simulink model "propeller"  (R2019b)
settings: Solver=VariableStepAuto  StartTime=0.0  StopTime=180  MaxStep=1e-2  RelTol=1e-3
undefined symbols (not defined in the file or in its folder): X, Y, Z
libraries: sm_lib x26, cstblocks x23, nesl_utility x20, simulink x2
(part 3 of 3)

== system propeller/直接转矩控制/船速、朝向控制器/推力解算/扭矩有解 ==
  状态输入 : Inport
  Action Port : ActionPort  ActionPortLabel=else
  If : If
  If Action Subsystem : Subsystem  TreatAsAtomicUnit=on
  If Action Subsystem1 : Subsystem  TreatAsAtomicUnit=on
  Merge : Merge
  通解选择 : Fcn  Expr=abs(u(5)+u(3)) - abs(u(5)-u(4))
  推力输出 : Outport
  wires:
  If Action Subsystem/1(推力) -> Merge/1
  If/1 -> If Action Subsystem/Action
  状态输入/1 -> If Action Subsystem1/1(In1), 通解选择/1, If Action Subsystem/1(In1)
  通解选择/1 -> If/1
  If Action Subsystem1/1(推力) -> Merge/2
  If/2 -> If Action Subsystem1/Action
  Merge/1 -> 推力输出/1  "推力输出"

== system propeller/直接转矩控制/船速、朝向控制器/舵内缩指令/If Action Subsystem ==
  Action Port : ActionPort  ActionPortLabel=else
  Constant : Constant  Value=0
  Out1 : Outport
  wires:
  Constant/1 -> Out1/1

== system propeller/直接转矩控制/船速、朝向控制器/舵内缩指令/Subsystem ==
  前进力 : Inport
  转向扭矩 : Inport  Port=2
  Action Port : ActionPort  ActionPortLabel=if(u1 < 0)
  Constant : Constant  Value=Trq_Start
  Gain : Gain  Gain=0.5
  Gain1 : Gain  Gain=0.1
  Gain2 : Gain  Gain=-1
  Integrator : Integrator  LimitOutput=on  UpperSaturationLimit=Th_Max*2  LowerSaturationLimit=0
  Mux : Mux  Inputs=2
  Sum : Sum  Inputs=|+-
  Sum3 : Sum  Inputs=|+-
  收敛用推力解算 : Subsystem  mask{a=1, b=3}
      mask prompts: a "推进器安装横向距离 a"; b "推进器安装纵向距离 b"
  左右差 : Outport
  wires:
  转向扭矩/1 -> 收敛用推力解算/2(转向扭矩)
  收敛用推力解算/1(左推力) -> Sum3/1
  Mux/1 -> 收敛用推力解算/3(左右推进偏角)
  Sum3/1 -> Sum/1
  前进力/1 -> 收敛用推力解算/1(前进力)
  Integrator/1 -> Gain/1, 左右差/1
  Gain/1 -> Gain2/1, Mux/1
  收敛用推力解算/2(右推力) -> Sum3/2
  Gain2/1 -> Mux/2
  Constant/1 -> Sum/2
  Sum/1 -> Gain1/1
  Gain1/1 -> Integrator/1

== system propeller/直接转矩控制/船速、朝向控制器/舵朝向指令/If Action Subsystem ==
  Action Port : ActionPort  ActionPortLabel=else
  Constant : Constant  Value=0
  Out1 : Outport
  wires:
  Constant/1 -> Out1/1

== system propeller/直接转矩控制/船速、朝向控制器/舵朝向指令/Subsystem ==
  前进力 : Inport
  转向扭矩 : Inport  Port=2
  Action Port : ActionPort  ActionPortLabel=if(u1 > 0)
  Gain : Gain  Gain=0.5
  Gain1 : Gain  Gain=0.1
  Integrator : Integrator  LimitOutput=on  UpperSaturationLimit=Th_Max*2  LowerSaturationLimit=-Th_Max*2
  Mux : Mux  Inputs=2
  Sum3 : Sum  Inputs=|+-
  收敛用推力解算 : Subsystem  mask{a=1, b=3}
      mask prompts: a "推进器安装横向距离 a"; b "推进器安装纵向距离 b"
  左右和 : Outport
  wires:
  收敛用推力解算/2(右推力) -> Sum3/2
  Gain/1 -> Mux/1, Mux/2
  Integrator/1 -> 左右和/1, Gain/1
  前进力/1 -> 收敛用推力解算/1(前进力)
  Sum3/1 -> Gain1/1
  Gain1/1 -> Integrator/1
  Mux/1 -> 收敛用推力解算/3(左右推进偏角)
  收敛用推力解算/1(左推力) -> Sum3/1
  转向扭矩/1 -> 收敛用推力解算/2(转向扭矩)

== system propeller/直接转矩控制/船速、朝向控制器/船头方向PID/反馈量滤波 ==
  Signal : Inport
  Constant2 : Constant  Value=Frq
  Gain : Gain  Gain=2*pi
  d_Smp_LPF6 : cstblocks/Linear Parameter Varying/Varying Lowpass Filter  N=Order
      settings: SourceProductName=Control System Toolbox
  Output : Outport
  wires:
  Gain/1 -> d_Smp_LPF6/2
  Signal/1 -> d_Smp_LPF6/1
  Constant2/1 -> Gain/1
  d_Smp_LPF6/1 -> Output/1  "Is"

== system propeller/直接转矩控制/船速、朝向控制器/船头方向PID/微分 ==
  Err : Inport
  Derivative : Derivative  CoefficientInTFapproximation=0.1
  微分滤波1 : Subsystem  mask{Frq=fc_Set, Order=3}
      mask prompts: Frq "Frq_Set"; Order "Order_Set"
  dErr : Outport
  wires:
  Err/1 -> 微分滤波1/1(Signal)
  微分滤波1/1(Output) -> Derivative/1
  Derivative/1 -> dErr/1

== system propeller/直接转矩控制/船速、朝向控制器/船头方向PID/积分控制 ==
  note: 角度快速增大时积分不增大
      | 角度快速减小时积分不减小
  Error : Inport
  Output : Inport  Port=2
  Derivative : Derivative  CoefficientInTFapproximation=0.1
  Memory : Memory
  Memory1 : Memory
  Product1 : Product  Inputs=3
  Scope : Scope  NumInputPorts=3
  Subsystem : Subsystem
  Zero-Order Hold : ZeroOrderHold  SampleTime=0.01
  Zero-Order Hold1 : ZeroOrderHold  SampleTime=0.01
  Zero-Order Hold2 : ZeroOrderHold  SampleTime=0.01
  输出达到正限幅时积分不再增大 : Subsystem
  输出达到负限幅时积分不再减小 : Subsystem
  开启积分 : Outport
  wires:
  Memory1/1 -> 输出达到正限幅时积分不再增大/2(Out), 输出达到负限幅时积分不再减小/2(Out)
  Memory/1 -> Subsystem/2(Err), 输出达到负限幅时积分不再减小/1(Err), 输出达到正限幅时积分不再增大/1(Err)
  Error/1 -> Derivative/1, Zero-Order Hold/1
  Product1/1 -> 开启积分/1
  Output/1 -> Zero-Order Hold2/1
  输出达到负限幅时积分不再减小/1(启动积分) -> Scope/3, Product1/3  "负限幅限制"
  输出达到正限幅时积分不再增大/1(启动积分) -> Scope/2, Product1/2  "正限幅限制"
  Zero-Order Hold/1 -> Memory/1
  Derivative/1 -> Zero-Order Hold1/1
  Zero-Order Hold2/1 -> Memory1/1
  Zero-Order Hold1/1 -> Subsystem/1(dErr)
  Subsystem/1(启动积分) -> Scope/1, Product1/1  "斜率限制"

== system propeller/失败的水流估计模型/水流状态估计/螺旋桨状态模拟/螺旋桨工作特性表/If Action Subsystem2 ==
  J' : Inport
  Action Port : ActionPort  ActionPortLabel=if(u1 > 0)
  n+::Kq-扭矩系数 : Lookup_n-D  NumberOfTableDimensions=1  BreakpointsForDimension1=[-1,-0.9,-0.8,-0.7,-0.6,-0.5,-0.4,-0.3,-0.2,-0.1,0,0.1,0.2,0.3,0.4,0.5,0.6,0.7,0.8,0.9,1]  BreakpointsForDimension2=[1:3]  Table=[0.019242,0.038636,0.046717,0.049444,0.050032,0.050032,0.050291,0.05055,0.051327,0.051845,0.05197,0.050556,0.046111,0.040556,0.033081,0.024596,0.015543,0.0059848,-0.0059091,-0.013687,-0.016818]  InternalRulePriority=Speed  RndMeth=Simplest  InputSameDT=on
  n+::Kt-推力系数 : Lookup_n-D  NumberOfTableDimensions=1  BreakpointsForDimension1=[-1,-0.9,-0.8,-0.7,-0.6,-0.5,-0.4,-0.3,-0.2,-0.1,0,0.1,0.2,0.3,0.4,0.5,0.6,0.7,0.8,0.9,1]  BreakpointsForDimension2=[1:3]  Table=[0.082134,0.19766,0.30499,0.32898,0.33608,0.33932,0.34256,0.34741,0.36197,0.3738,0.38,0.36686,0.32645,0.26016,0.18188,0.10423,0.04173,-0.018245,-0.05423,-0.065593,-0.06]  InternalRulePriority=Speed  RndMeth=Simplest  InputSameDT=on
  Kt : Outport
  Kq : Outport  Port=2
  wires:
  J'/1 -> n+::Kt-推力系数/1, n+::Kq-扭矩系数/1
  n+::Kt-推力系数/1 -> Kt/1
  n+::Kq-扭矩系数/1 -> Kq/1

== system propeller/失败的水流估计模型/水流状态估计/螺旋桨状态模拟/螺旋桨工作特性表/If Action Subsystem3 ==
  J' : Inport
  Action Port : ActionPort  ActionPortLabel=else
  n-::Kq-扭矩系数 : Lookup_n-D  NumberOfTableDimensions=1  BreakpointsForDimension1=[-1,-0.9,-0.8,-0.7,-0.6,-0.5,-0.4,-0.3,-0.2,-0.1,0,0.1,0.2,0.3,0.4,0.5,0.6,0.7,0.8,0.9,1]  BreakpointsForDimension2=[1:3]  Table=[0.019242,0.016111,0.010354,-0.00035354,-0.014293,-0.025707,-0.034495,-0.041263,-0.046515,-0.051162,-0.05197,-0.051845,-0.051586,-0.051068,-0.051068,-0.050809,-0.050291,-0.048997,-0.045631,-0.038434,-0.016818]  InternalRulePriority=Speed  RndMeth=Simplest  InputSameDT=on
  n-::Kt-推力系数 : Lookup_n-D  NumberOfTableDimensions=1  BreakpointsForDimension1=[-1,-0.9,-0.8,-0.7,-0.6,-0.5,-0.4,-0.3,-0.2,-0.1,0,0.1,0.2,0.3,0.4,0.5,0.6,0.7,0.8,0.9,1]  BreakpointsForDimension2=[1:3]  Table=[0.082134,0.088952,0.080745,0.052336,-0.020896,-0.090341,-0.16989,-0.25764,-0.32014,-0.34981,-0.35874,-0.36197,-0.36036,-0.35874,-0.35388,-0.34741,-0.3377,-0.32197,-0.2947,-0.21894,-0.06]  InternalRulePriority=Speed  RndMeth=Simplest  InputSameDT=on
  Kt : Outport
  Kq : Outport  Port=2
  wires:
  n-::Kq-扭矩系数/1 -> Kq/1
  n-::Kt-推力系数/1 -> Kt/1
  J'/1 -> n-::Kt-推力系数/1, n-::Kq-扭矩系数/1

== system propeller/失败的水流估计模型/水流状态估计/螺旋桨状态模拟/螺旋桨工作特性表Backup/If Action Subsystem2 ==
  J' : Inport
  Action Port : ActionPort
  n+::Kq-扭矩系数 : Lookup_n-D  NumberOfTableDimensions=1  BreakpointsForDimension1=[-1,-0.9,-0.8,-0.7,-0.6,-0.5,-0.4,-0.3,-0.2,-0.1,0,0.1,0.2,0.3,0.4,0.5,0.6,0.7,0.8,0.9,1]  BreakpointsForDimension2=[1:3]  Table=[0.019242,0.038636,0.046717,0.049444,0.048333,0.043384,0.043081,0.045202,0.049242,0.051465,0.05197,0.050556,0.046111,0.040556,0.033081,0.024596,0.015543,0.0059848,-0.0059091,-0.013687,-0.016818]  InternalRulePriority=Speed  RndMeth=Simplest  InputSameDT=on
  n+::Kt-推力系数 : Lookup_n-D  NumberOfTableDimensions=1  BreakpointsForDimension1=[-1,-0.9,-0.8,-0.7,-0.6,-0.5,-0.4,-0.3,-0.2,-0.1,0,0.1,0.2,0.3,0.4,0.5,0.6,0.7,0.8,0.9,1]  BreakpointsForDimension2=[1:3]  Table=[0.082134,0.19766,0.30499,0.32898,0.31256,0.2589,0.25511,0.28226,0.35107,0.3738,0.38,0.36686,0.32645,0.26016,0.18188,0.10423,0.04173,-0.018245,-0.05423,-0.065593,-0.06]  InternalRulePriority=Speed  RndMeth=Simplest  InputSameDT=on
  Kt : Outport
  Kq : Outport  Port=2
  wires:
  n+::Kq-扭矩系数/1 -> Kq/1
  n+::Kt-推力系数/1 -> Kt/1
  J'/1 -> n+::Kq-扭矩系数/1, n+::Kt-推力系数/1

== system propeller/失败的水流估计模型/水流状态估计/螺旋桨状态模拟/螺旋桨工作特性表Backup/If Action Subsystem3 ==
  J' : Inport
  Action Port : ActionPort
  n-::Kq-扭矩系数 : Lookup_n-D  NumberOfTableDimensions=1  BreakpointsForDimension1=[-1,-0.9,-0.8,-0.7,-0.6,-0.5,-0.4,-0.3,-0.2,-0.1,0,0.1,0.2,0.3,0.4,0.5,0.6,0.7,0.8,0.9,1]  BreakpointsForDimension2=[1:3]  Table=[0.019242,0.016111,0.010354,-0.00035354,-0.014293,-0.025707,-0.034495,-0.041263,-0.046515,-0.051162,-0.05197,-0.051465,-0.049242,-0.045202,-0.043081,-0.043384,-0.04702,-0.049343,-0.045909,-0.038434,-0.016818]  InternalRulePriority=Speed  RndMeth=Simplest  InputSameDT=on
  n-::Kt-推力系数 : Lookup_n-D  NumberOfTableDimensions=1  BreakpointsForDimension1=[-1,-0.9,-0.8,-0.7,-0.6,-0.5,-0.4,-0.3,-0.2,-0.1,0,0.1,0.2,0.3,0.4,0.5,0.6,0.7,0.8,0.9,1]  BreakpointsForDimension2=[1:3]  Table=[0.082134,0.088952,0.080745,0.052336,-0.020896,-0.090341,-0.16989,-0.25764,-0.32014,-0.34981,-0.35676,-0.35549,-0.33409,-0.29015,-0.25379,-0.24924,-0.30379,-0.32197,-0.2947,-0.21894,-0.06]  InternalRulePriority=Speed  RndMeth=Simplest  InputSameDT=on
  Kt : Outport
  Kq : Outport  Port=2
  wires:
  J'/1 -> n-::Kq-扭矩系数/1, n-::Kt-推力系数/1
  n-::Kt-推力系数/1 -> Kt/1
  n-::Kq-扭矩系数/1 -> Kq/1

== system propeller/失败的水流估计模型/预期转速计算/螺旋桨状态模拟/螺旋桨工作特性表/If Action Subsystem2 ==
  J' : Inport
  Action Port : ActionPort  ActionPortLabel=if(u1 > 0)
  n+::Kq-扭矩系数 : Lookup_n-D  NumberOfTableDimensions=1  BreakpointsForDimension1=[-1,-0.9,-0.8,-0.7,-0.6,-0.5,-0.4,-0.3,-0.2,-0.1,0,0.1,0.2,0.3,0.4,0.5,0.6,0.7,0.8,0.9,1]  BreakpointsForDimension2=[1:3]  Table=[0.019242,0.038636,0.046717,0.049444,0.050032,0.050032,0.050291,0.05055,0.051327,0.051845,0.05197,0.050556,0.046111,0.040556,0.033081,0.024596,0.015543,0.0059848,-0.0059091,-0.013687,-0.016818]  InternalRulePriority=Speed  RndMeth=Simplest  InputSameDT=on
  n+::Kt-推力系数 : Lookup_n-D  NumberOfTableDimensions=1  BreakpointsForDimension1=[-1,-0.9,-0.8,-0.7,-0.6,-0.5,-0.4,-0.3,-0.2,-0.1,0,0.1,0.2,0.3,0.4,0.5,0.6,0.7,0.8,0.9,1]  BreakpointsForDimension2=[1:3]  Table=[0.082134,0.19766,0.30499,0.32898,0.33608,0.33932,0.34256,0.34741,0.36197,0.3738,0.38,0.36686,0.32645,0.26016,0.18188,0.10423,0.04173,-0.018245,-0.05423,-0.065593,-0.06]  InternalRulePriority=Speed  RndMeth=Simplest  InputSameDT=on
  Kt : Outport
  Kq : Outport  Port=2
  wires:
  J'/1 -> n+::Kt-推力系数/1, n+::Kq-扭矩系数/1
  n+::Kt-推力系数/1 -> Kt/1
  n+::Kq-扭矩系数/1 -> Kq/1

== system propeller/失败的水流估计模型/预期转速计算/螺旋桨状态模拟/螺旋桨工作特性表/If Action Subsystem3 ==
  J' : Inport
  Action Port : ActionPort  ActionPortLabel=else
  n-::Kq-扭矩系数 : Lookup_n-D  NumberOfTableDimensions=1  BreakpointsForDimension1=[-1,-0.9,-0.8,-0.7,-0.6,-0.5,-0.4,-0.3,-0.2,-0.1,0,0.1,0.2,0.3,0.4,0.5,0.6,0.7,0.8,0.9,1]  BreakpointsForDimension2=[1:3]  Table=[0.019242,0.016111,0.010354,-0.00035354,-0.014293,-0.025707,-0.034495,-0.041263,-0.046515,-0.051162,-0.05197,-0.051845,-0.051586,-0.051068,-0.051068,-0.050809,-0.050291,-0.048997,-0.045631,-0.038434,-0.016818]  InternalRulePriority=Speed  RndMeth=Simplest  InputSameDT=on
  n-::Kt-推力系数 : Lookup_n-D  NumberOfTableDimensions=1  BreakpointsForDimension1=[-1,-0.9,-0.8,-0.7,-0.6,-0.5,-0.4,-0.3,-0.2,-0.1,0,0.1,0.2,0.3,0.4,0.5,0.6,0.7,0.8,0.9,1]  BreakpointsForDimension2=[1:3]  Table=[0.082134,0.088952,0.080745,0.052336,-0.020896,-0.090341,-0.16989,-0.25764,-0.32014,-0.34981,-0.35874,-0.36197,-0.36036,-0.35874,-0.35388,-0.34741,-0.3377,-0.32197,-0.2947,-0.21894,-0.06]  InternalRulePriority=Speed  RndMeth=Simplest  InputSameDT=on
  Kt : Outport
  Kq : Outport  Port=2
  wires:
  n-::Kq-扭矩系数/1 -> Kq/1
  n-::Kt-推力系数/1 -> Kt/1
  J'/1 -> n-::Kt-推力系数/1, n-::Kq-扭矩系数/1

== system propeller/失败的水流估计模型/预期转速计算/螺旋桨状态模拟/螺旋桨工作特性表Backup/If Action Subsystem2 ==
  J' : Inport
  Action Port : ActionPort
  n+::Kq-扭矩系数 : Lookup_n-D  NumberOfTableDimensions=1  BreakpointsForDimension1=[-1,-0.9,-0.8,-0.7,-0.6,-0.5,-0.4,-0.3,-0.2,-0.1,0,0.1,0.2,0.3,0.4,0.5,0.6,0.7,0.8,0.9,1]  BreakpointsForDimension2=[1:3]  Table=[0.019242,0.038636,0.046717,0.049444,0.048333,0.043384,0.043081,0.045202,0.049242,0.051465,0.05197,0.050556,0.046111,0.040556,0.033081,0.024596,0.015543,0.0059848,-0.0059091,-0.013687,-0.016818]  InternalRulePriority=Speed  RndMeth=Simplest  InputSameDT=on
  n+::Kt-推力系数 : Lookup_n-D  NumberOfTableDimensions=1  BreakpointsForDimension1=[-1,-0.9,-0.8,-0.7,-0.6,-0.5,-0.4,-0.3,-0.2,-0.1,0,0.1,0.2,0.3,0.4,0.5,0.6,0.7,0.8,0.9,1]  BreakpointsForDimension2=[1:3]  Table=[0.082134,0.19766,0.30499,0.32898,0.31256,0.2589,0.25511,0.28226,0.35107,0.3738,0.38,0.36686,0.32645,0.26016,0.18188,0.10423,0.04173,-0.018245,-0.05423,-0.065593,-0.06]  InternalRulePriority=Speed  RndMeth=Simplest  InputSameDT=on
  Kt : Outport
  Kq : Outport  Port=2
  wires:
  n+::Kq-扭矩系数/1 -> Kq/1
  n+::Kt-推力系数/1 -> Kt/1
  J'/1 -> n+::Kq-扭矩系数/1, n+::Kt-推力系数/1

== system propeller/失败的水流估计模型/预期转速计算/螺旋桨状态模拟/螺旋桨工作特性表Backup/If Action Subsystem3 ==
  J' : Inport
  Action Port : ActionPort
  n-::Kq-扭矩系数 : Lookup_n-D  NumberOfTableDimensions=1  BreakpointsForDimension1=[-1,-0.9,-0.8,-0.7,-0.6,-0.5,-0.4,-0.3,-0.2,-0.1,0,0.1,0.2,0.3,0.4,0.5,0.6,0.7,0.8,0.9,1]  BreakpointsForDimension2=[1:3]  Table=[0.019242,0.016111,0.010354,-0.00035354,-0.014293,-0.025707,-0.034495,-0.041263,-0.046515,-0.051162,-0.05197,-0.051465,-0.049242,-0.045202,-0.043081,-0.043384,-0.04702,-0.049343,-0.045909,-0.038434,-0.016818]  InternalRulePriority=Speed  RndMeth=Simplest  InputSameDT=on
  n-::Kt-推力系数 : Lookup_n-D  NumberOfTableDimensions=1  BreakpointsForDimension1=[-1,-0.9,-0.8,-0.7,-0.6,-0.5,-0.4,-0.3,-0.2,-0.1,0,0.1,0.2,0.3,0.4,0.5,0.6,0.7,0.8,0.9,1]  BreakpointsForDimension2=[1:3]  Table=[0.082134,0.088952,0.080745,0.052336,-0.020896,-0.090341,-0.16989,-0.25764,-0.32014,-0.34981,-0.35676,-0.35549,-0.33409,-0.29015,-0.25379,-0.24924,-0.30379,-0.32197,-0.2947,-0.21894,-0.06]  InternalRulePriority=Speed  RndMeth=Simplest  InputSameDT=on
  Kt : Outport
  Kq : Outport  Port=2
  wires:
  J'/1 -> n-::Kq-扭矩系数/1, n-::Kt-推力系数/1
  n-::Kt-推力系数/1 -> Kt/1
  n-::Kq-扭矩系数/1 -> Kq/1

== system propeller/直接转矩控制/船体、水体物理模型/推进器1/螺旋桨模型/If Action Subsystem ==
  In1 : Inport
  Action Port : ActionPort  ActionPortLabel=else
  Fcn2 : Fcn  Expr=u(1)/(sqrt(u(2)))
  Out1 : Outport
  wires:
  Fcn2/1 -> Out1/1
  In1/1 -> Fcn2/1

== system propeller/直接转矩控制/船体、水体物理模型/推进器1/螺旋桨模型/If Action Subsystem1 ==
  In1 : Inport
  Action Port : ActionPort  ActionPortLabel=if(u1 < 1e-6)
  Fcn2 : Fcn  Expr=abs(u(1))
  Out1 : Outport
  wires:
  In1/1 -> Fcn2/1
  Fcn2/1 -> Out1/1

== system propeller/直接转矩控制/船体、水体物理模型/推进器1/螺旋桨模型/螺旋桨工作特性表 ==
  J' : Inport
  转速 : Inport  Port=2
  If Action Subsystem2 : Subsystem  TreatAsAtomicUnit=on
  If Action Subsystem3 : Subsystem  TreatAsAtomicUnit=on
  If1 : If
  Merge1 : Merge
  Merge2 : Merge
  Kt : Outport
  Kq : Outport  Port=2
  wires:
  If Action Subsystem2/2(Kq) -> Merge2/1
  Merge2/1 -> Kq/1
  If Action Subsystem3/2(Kq) -> Merge2/2
  If Action Subsystem3/1(Kt) -> Merge1/2
  Merge1/1 -> Kt/1
  J'/1 -> If Action Subsystem2/1(J'), If Action Subsystem3/1(J')
  If Action Subsystem2/1(Kt) -> Merge1/1
  转速/1 -> If1/1
  If1/2 -> If Action Subsystem3/Action
  If1/1 -> If Action Subsystem2/Action

== system propeller/直接转矩控制/船体、水体物理模型/推进器1/螺旋桨模型/螺旋桨工作特性表Backup ==
  J' : Inport
  转速 : Inport  Port=2
  If Action Subsystem2 : Subsystem  TreatAsAtomicUnit=on
  If Action Subsystem3 : Subsystem  TreatAsAtomicUnit=on
  If1 : If
  Merge1 : Merge
  Merge2 : Merge
  Kt : Outport
  Kq : Outport  Port=2
  wires:
  If1/1 -> If Action Subsystem2/Action
  If1/2 -> If Action Subsystem3/Action
  转速/1 -> If1/1
  If Action Subsystem2/1(Kt) -> Merge1/1
  J'/1 -> If Action Subsystem3/1(J'), If Action Subsystem2/1(J')
  Merge1/1 -> Kt/1
  If Action Subsystem3/1(Kt) -> Merge1/2
  If Action Subsystem3/2(Kq) -> Merge2/2
  Merge2/1 -> Kq/1
  If Action Subsystem2/2(Kq) -> Merge2/1

== system propeller/直接转矩控制/船体、水体物理模型/推进器1/驱动电机/反馈量滤波 ==
  Signal : Inport
  Constant2 : Constant  Value=Frq
  Gain : Gain  Gain=2*pi
  d_Smp_LPF6 : cstblocks/Linear Parameter Varying/Varying Lowpass Filter  N=Order
      settings: SourceProductName=Control System Toolbox
  Output : Outport
  wires:
  d_Smp_LPF6/1 -> Output/1  "Is"
  Constant2/1 -> Gain/1
  Signal/1 -> d_Smp_LPF6/1
  Gain/1 -> d_Smp_LPF6/2

== system propeller/直接转矩控制/船体、水体物理模型/推进器1/驱动电机/滞后 ==
  Signal : Inport
  Constant2 : Constant  Value=Frq
  Gain : Gain  Gain=2*pi
  d_Smp_LPF6 : cstblocks/Linear Parameter Varying/Varying Lowpass Filter  N=Order
      settings: SourceProductName=Control System Toolbox
  Output : Outport
  wires:
  d_Smp_LPF6/1 -> Output/1  "Is"
  Constant2/1 -> Gain/1
  Signal/1 -> d_Smp_LPF6/1
  Gain/1 -> d_Smp_LPF6/2

== system propeller/直接转矩控制/船体、水体物理模型/推进器2/螺旋桨模型/If Action Subsystem ==
  In1 : Inport
  Action Port : ActionPort  ActionPortLabel=else
  Fcn2 : Fcn  Expr=u(1)/(sqrt(u(2)))
  Out1 : Outport
  wires:
  In1/1 -> Fcn2/1
  Fcn2/1 -> Out1/1

== system propeller/直接转矩控制/船体、水体物理模型/推进器2/螺旋桨模型/If Action Subsystem1 ==
  In1 : Inport
  Action Port : ActionPort  ActionPortLabel=if(u1 < 1e-6)
  Fcn2 : Fcn  Expr=abs(u(1))
  Out1 : Outport
  wires:
  Fcn2/1 -> Out1/1
  In1/1 -> Fcn2/1

== system propeller/直接转矩控制/船体、水体物理模型/推进器2/螺旋桨模型/螺旋桨工作特性表 ==
  J' : Inport
  转速 : Inport  Port=2
  If Action Subsystem2 : Subsystem  TreatAsAtomicUnit=on
  If Action Subsystem3 : Subsystem  TreatAsAtomicUnit=on
  If1 : If
  Merge1 : Merge
  Merge2 : Merge
  Kt : Outport
  Kq : Outport  Port=2
  wires:
  If1/1 -> If Action Subsystem2/Action
  If1/2 -> If Action Subsystem3/Action
  转速/1 -> If1/1
  If Action Subsystem2/1(Kt) -> Merge1/1
  J'/1 -> If Action Subsystem3/1(J'), If Action Subsystem2/1(J')
  Merge1/1 -> Kt/1
  If Action Subsystem3/1(Kt) -> Merge1/2
  If Action Subsystem3/2(Kq) -> Merge2/2
  Merge2/1 -> Kq/1
  If Action Subsystem2/2(Kq) -> Merge2/1

== system propeller/直接转矩控制/船体、水体物理模型/推进器2/螺旋桨模型/螺旋桨工作特性表Backup ==
  J' : Inport
  转速 : Inport  Port=2
  If Action Subsystem2 : Subsystem  TreatAsAtomicUnit=on
  If Action Subsystem3 : Subsystem  TreatAsAtomicUnit=on
  If1 : If
  Merge1 : Merge
  Merge2 : Merge
  Kt : Outport
  Kq : Outport  Port=2
  wires:
  If Action Subsystem2/2(Kq) -> Merge2/1
  Merge2/1 -> Kq/1
  If Action Subsystem3/2(Kq) -> Merge2/2
  If Action Subsystem3/1(Kt) -> Merge1/2
  Merge1/1 -> Kt/1
  J'/1 -> If Action Subsystem2/1(J'), If Action Subsystem3/1(J')
  If Action Subsystem2/1(Kt) -> Merge1/1
  转速/1 -> If1/1
  If1/2 -> If Action Subsystem3/Action
  If1/1 -> If Action Subsystem2/Action

== system propeller/直接转矩控制/船体、水体物理模型/推进器2/驱动电机/反馈量滤波 ==
  Signal : Inport
  Constant2 : Constant  Value=Frq
  Gain : Gain  Gain=2*pi
  d_Smp_LPF6 : cstblocks/Linear Parameter Varying/Varying Lowpass Filter  N=Order
      settings: SourceProductName=Control System Toolbox
  Output : Outport
  wires:
  Gain/1 -> d_Smp_LPF6/2
  Signal/1 -> d_Smp_LPF6/1
  Constant2/1 -> Gain/1
  d_Smp_LPF6/1 -> Output/1  "Is"

== system propeller/直接转矩控制/船体、水体物理模型/推进器2/驱动电机/滞后 ==
  Signal : Inport
  Constant2 : Constant  Value=Frq
  Gain : Gain  Gain=2*pi
  d_Smp_LPF6 : cstblocks/Linear Parameter Varying/Varying Lowpass Filter  N=Order
      settings: SourceProductName=Control System Toolbox
  Output : Outport
  wires:
  Gain/1 -> d_Smp_LPF6/2
  Signal/1 -> d_Smp_LPF6/1
  Constant2/1 -> Gain/1
  d_Smp_LPF6/1 -> Output/1  "Is"

== system propeller/直接转矩控制/船速、朝向控制器/前进速度控制/微分/微分滤波1 ==
  Signal : Inport
  Constant2 : Constant  Value=Frq
  Gain : Gain  Gain=2*pi
  d_Smp_LPF6 : cstblocks/Linear Parameter Varying/Varying Lowpass Filter  N=Order
      settings: SourceProductName=Control System Toolbox
  Output : Outport
  wires:
  d_Smp_LPF6/1 -> Output/1  "Is"
  Constant2/1 -> Gain/1
  Signal/1 -> d_Smp_LPF6/1
  Gain/1 -> d_Smp_LPF6/2

== system propeller/直接转矩控制/船速、朝向控制器/前进速度控制/积分控制/Subsystem ==
  dErr : Inport
  Err : Inport  Port=2
  Abs : Abs
  Constant10 : Constant
  Constant3 : Constant  Value=0
  Constant4 : Constant
  Memory2 : Memory
  Product : Product
  Switch1 : Switch  Criteria=u2 > Threshold  Threshold=dSpe
  Switch6 : Switch  Criteria=u2 > Threshold
  启动积分 : Outport
  wires:
  Switch1/1 -> 启动积分/1
  Err/1 -> Product/2
  Switch6/1 -> Switch1/1
  Product/1 -> Memory2/1
  Constant3/1 -> Switch6/3
  Abs/1 -> Switch1/2
  Constant4/1 -> Switch1/3
  Constant10/1 -> Switch6/1
  dErr/1 -> Abs/1, Product/1
  Memory2/1 -> Switch6/2

== system propeller/直接转矩控制/船速、朝向控制器/前进速度控制/积分控制/输出达到正限幅时积分不再增大 ==
  Err : Inport
  Out : Inport  Port=2
  Constant : Constant  Value=Trq_p
  Constant2 : Constant
  Constant5 : Constant  Value=0
  Constant6 : Constant
  Sum2 : Sum  Inputs=-+|
  Switch2 : Switch  Criteria=u2 > Threshold
  Switch3 : Switch  Criteria=u2 > Threshold
  启动积分 : Outport
  wires:
  Err/1 -> Switch2/2
  Switch3/1 -> Switch2/1
  Constant/1 -> Sum2/1
  Constant2/1 -> Switch2/3
  Constant6/1 -> Switch3/3
  Out/1 -> Sum2/2
  Sum2/1 -> Switch3/2
  Switch2/1 -> 启动积分/1
  Constant5/1 -> Switch3/1

== system propeller/直接转矩控制/船速、朝向控制器/前进速度控制/积分控制/输出达到负限幅时积分不再减小 ==
  Err : Inport
  Out : Inport  Port=2
  Constant1 : Constant
  Constant7 : Constant  Value=0
  Constant8 : Constant
  Constant9 : Constant  Value=-Trq_n
  Sum3 : Sum  Inputs=+-|
  Switch4 : Switch  Criteria=u2 > Threshold
  Switch5 : Switch  Criteria=u2 > Threshold
  启动积分 : Outport
  wires:
  Constant8/1 -> Switch5/3
  Switch4/1 -> 启动积分/1
  Constant7/1 -> Switch5/1
  Constant9/1 -> Sum3/1
  Constant1/1 -> Switch4/1
  Err/1 -> Switch4/2
  Out/1 -> Sum3/2
  Switch5/1 -> Switch4/3
  Sum3/1 -> Switch5/2

== system propeller/直接转矩控制/船速、朝向控制器/右电机控制/角加速度补偿/滞后1 ==
  Signal : Inport
  Constant2 : Constant  Value=Frq
  Gain : Gain  Gain=2*pi
  d_Smp_LPF6 : cstblocks/Linear Parameter Varying/Varying Lowpass Filter  N=Order
      settings: SourceProductName=Control System Toolbox
  Output : Outport
  wires:
  Gain/1 -> d_Smp_LPF6/2
  Signal/1 -> d_Smp_LPF6/1
  Constant2/1 -> Gain/1
  d_Smp_LPF6/1 -> Output/1  "Is"

== system propeller/直接转矩控制/船速、朝向控制器/右电机控制/角加速度补偿/滞后2 ==
  Signal : Inport
  Constant2 : Constant  Value=Frq
  Gain : Gain  Gain=2*pi
  d_Smp_LPF6 : cstblocks/Linear Parameter Varying/Varying Lowpass Filter  N=Order
      settings: SourceProductName=Control System Toolbox
  Output : Outport
  wires:
  d_Smp_LPF6/1 -> Output/1  "Is"
  Constant2/1 -> Gain/1
  Signal/1 -> d_Smp_LPF6/1
  Gain/1 -> d_Smp_LPF6/2

== system propeller/直接转矩控制/船速、朝向控制器/左电机控制/角加速度补偿/滞后1 ==
  Signal : Inport
  Constant2 : Constant  Value=Frq
  Gain : Gain  Gain=2*pi
  d_Smp_LPF6 : cstblocks/Linear Parameter Varying/Varying Lowpass Filter  N=Order
      settings: SourceProductName=Control System Toolbox
  Output : Outport
  wires:
  d_Smp_LPF6/1 -> Output/1  "Is"
  Constant2/1 -> Gain/1
  Signal/1 -> d_Smp_LPF6/1
  Gain/1 -> d_Smp_LPF6/2

== system propeller/直接转矩控制/船速、朝向控制器/左电机控制/角加速度补偿/滞后2 ==
  Signal : Inport
  Constant2 : Constant  Value=Frq
  Gain : Gain  Gain=2*pi
  d_Smp_LPF6 : cstblocks/Linear Parameter Varying/Varying Lowpass Filter  N=Order
      settings: SourceProductName=Control System Toolbox
  Output : Outport
  wires:
  Gain/1 -> d_Smp_LPF6/2
  Signal/1 -> d_Smp_LPF6/1
  Constant2/1 -> Gain/1
  d_Smp_LPF6/1 -> Output/1  "Is"

== system propeller/直接转矩控制/船速、朝向控制器/推力解算/扭矩有解/If Action Subsystem ==
  In1 : Inport
  Action Port : ActionPort  ActionPortLabel=if(u1 > 0)
  Abs : Abs
  If : If  IfExpression=u1 < 1e-6
  Merge : Merge
  无解 : Subsystem  TreatAsAtomicUnit=on
  有解 : Subsystem  TreatAsAtomicUnit=on
  通解分母 : Fcn  Expr=(cos(u(4))/cos(u(3)) + sin(u(5)-u(4))/sin(u(5)+u(3)))
  推力 : Outport
  wires:
  通解分母/1 -> Abs/1
  In1/1 -> 有解/1(In1), 通解分母/1
  Abs/1 -> If/1
  If/1 -> 无解/Action
  If/2 -> 有解/Action
  Merge/1 -> 推力/1
  无解/1(Out1) -> Merge/1
  有解/1(Out1) -> Merge/2

== system propeller/直接转矩控制/船速、朝向控制器/推力解算/扭矩有解/If Action Subsystem1 ==
  In1 : Inport
  Action Port : ActionPort  ActionPortLabel=else
  Abs : Abs
  If : If  IfExpression=u1 < 1e-6
  Merge : Merge
  无解 : Subsystem  TreatAsAtomicUnit=on
  有解 : Subsystem  TreatAsAtomicUnit=on
  通解分母 : Fcn  Expr=(cos(u(3))/cos(u(4)) + sin(u(5)+u(3))/sin(u(5)-u(4)))
  推力 : Outport
  wires:
  有解/1(Out1) -> Merge/2
  无解/1(Out1) -> Merge/1
  Merge/1 -> 推力/1
  If/2 -> 有解/Action
  If/1 -> 无解/Action
  Abs/1 -> If/1
  In1/1 -> 通解分母/1, 有解/1(In1)
  通解分母/1 -> Abs/1

== system propeller/直接转矩控制/船速、朝向控制器/舵内缩指令/Subsystem/收敛用推力解算 ==
  前进力 : Inport
  转向扭矩 : Inport  Port=2
  左右推进偏角 : Inport  Port=3
  Demux : Demux  Outputs=2
  Demux1 : Demux  Outputs=2
  If1 : If  IfExpression=u1 < 1e-6
  Merge : Merge
  Mux : Mux  Inputs=6
  Th0 : Constant  Value=atan(a/b)
  c : Constant  Value=sqrt(a^2+b^2)
  扭矩无解 : Subsystem  TreatAsAtomicUnit=on
  扭矩无解检查 : Fcn  Expr=abs(u(5)+u(3)) + abs(u(5)-u(4))
  扭矩有解 : Subsystem
  左推力 : Outport
  右推力 : Outport  Port=2
  wires:
  前进力/1 -> Mux/1
  转向扭矩/1 -> Mux/2
  Demux/1 -> 左推力/1
  Demux/2 -> 右推力/1
  Demux1/2 -> Mux/4
  Demux1/1 -> Mux/3
  左右推进偏角/1 -> Demux1/1
  c/1 -> Mux/6
  Th0/1 -> Mux/5
  Merge/1 -> Demux/1
  扭矩无解检查/1 -> If1/1
  Mux/1 -> 扭矩有解/1(状态输入), 扭矩无解/1(In1), 扭矩无解检查/1  "状态输入"
  If1/1 -> 扭矩无解/Action
  If1/2 -> 扭矩有解/Action
  扭矩无解/1(Out1) -> Merge/1
  扭矩有解/1(推力输出) -> Merge/2

== system propeller/直接转矩控制/船速、朝向控制器/舵朝向指令/Subsystem/收敛用推力解算 ==
  前进力 : Inport
  转向扭矩 : Inport  Port=2
  左右推进偏角 : Inport  Port=3
  Demux : Demux  Outputs=2
  Demux1 : Demux  Outputs=2
  If1 : If  IfExpression=u1 < 1e-6
  Merge : Merge
  Mux : Mux  Inputs=6
  Th0 : Constant  Value=atan(a/b)
  c : Constant  Value=sqrt(a^2+b^2)
  扭矩无解 : Subsystem  TreatAsAtomicUnit=on
  扭矩无解检查 : Fcn  Expr=abs(u(5)+u(3)) + abs(u(5)-u(4))
  扭矩有解 : Subsystem
  左推力 : Outport
  右推力 : Outport  Port=2
  wires:
  扭矩有解/1(推力输出) -> Merge/2
  扭矩无解/1(Out1) -> Merge/1
  If1/2 -> 扭矩有解/Action
  If1/1 -> 扭矩无解/Action
  Mux/1 -> 扭矩无解检查/1, 扭矩无解/1(In1), 扭矩有解/1(状态输入)  "状态输入"
  扭矩无解检查/1 -> If1/1
  Merge/1 -> Demux/1
  Th0/1 -> Mux/5
  c/1 -> Mux/6
  左右推进偏角/1 -> Demux1/1
  Demux1/1 -> Mux/3
  Demux1/2 -> Mux/4
  Demux/2 -> 右推力/1
  Demux/1 -> 左推力/1
  转向扭矩/1 -> Mux/2
  前进力/1 -> Mux/1

== system propeller/直接转矩控制/船速、朝向控制器/船头方向PID/微分/微分滤波1 ==
  Signal : Inport
  Constant2 : Constant  Value=Frq
  Gain : Gain  Gain=2*pi
  d_Smp_LPF6 : cstblocks/Linear Parameter Varying/Varying Lowpass Filter  N=Order
      settings: SourceProductName=Control System Toolbox
  Output : Outport
  wires:
  Gain/1 -> d_Smp_LPF6/2
  Signal/1 -> d_Smp_LPF6/1
  Constant2/1 -> Gain/1
  d_Smp_LPF6/1 -> Output/1  "Is"

== system propeller/直接转矩控制/船速、朝向控制器/船头方向PID/积分控制/Subsystem ==
  dErr : Inport
  Err : Inport  Port=2
  Abs : Abs
  Constant10 : Constant
  Constant3 : Constant  Value=0
  Constant4 : Constant
  Memory2 : Memory
  Product : Product
  Switch1 : Switch  Criteria=u2 > Threshold  Threshold=dAng
  Switch6 : Switch  Criteria=u2 > Threshold
  启动积分 : Outport
  wires:
  Memory2/1 -> Switch6/2
  dErr/1 -> Product/1, Abs/1
  Constant10/1 -> Switch6/1
  Constant4/1 -> Switch1/3
  Abs/1 -> Switch1/2
  Constant3/1 -> Switch6/3
  Product/1 -> Memory2/1
  Switch6/1 -> Switch1/1
  Err/1 -> Product/2
  Switch1/1 -> 启动积分/1

== system propeller/直接转矩控制/船速、朝向控制器/船头方向PID/积分控制/输出达到正限幅时积分不再增大 ==
  Err : Inport
  Out : Inport  Port=2
  Constant : Constant  Value=Spe_p
  Constant2 : Constant
  Constant5 : Constant  Value=0
  Constant6 : Constant
  Sum2 : Sum  Inputs=-+|
  Switch2 : Switch  Criteria=u2 > Threshold
  Switch3 : Switch  Criteria=u2 > Threshold
  启动积分 : Outport
  wires:
  Constant5/1 -> Switch3/1
  Switch2/1 -> 启动积分/1
  Sum2/1 -> Switch3/2
  Out/1 -> Sum2/2
  Constant6/1 -> Switch3/3
  Constant2/1 -> Switch2/3
  Constant/1 -> Sum2/1
  Switch3/1 -> Switch2/1
  Err/1 -> Switch2/2

== system propeller/直接转矩控制/船速、朝向控制器/船头方向PID/积分控制/输出达到负限幅时积分不再减小 ==
  Err : Inport
  Out : Inport  Port=2
  Constant1 : Constant
  Constant7 : Constant  Value=0
  Constant8 : Constant
  Constant9 : Constant  Value=-Spe_n
  Sum3 : Sum  Inputs=+-|
  Switch4 : Switch  Criteria=u2 > Threshold
  Switch5 : Switch  Criteria=u2 > Threshold
  启动积分 : Outport
  wires:
  Sum3/1 -> Switch5/2
  Switch5/1 -> Switch4/3
  Out/1 -> Sum3/2
  Err/1 -> Switch4/2
  Constant1/1 -> Switch4/1
  Constant9/1 -> Sum3/1
  Constant7/1 -> Switch5/1
  Switch4/1 -> 启动积分/1
  Constant8/1 -> Switch5/3

== system propeller/直接转矩控制/船体、水体物理模型/推进器1/螺旋桨模型/螺旋桨工作特性表/If Action Subsystem2 ==
  J' : Inport
  Action Port : ActionPort  ActionPortLabel=if(u1 > 0)
  n+::Kq-扭矩系数 : Lookup_n-D  NumberOfTableDimensions=1  BreakpointsForDimension1=[-1,-0.9,-0.8,-0.7,-0.6,-0.5,-0.4,-0.3,-0.2,-0.1,0,0.1,0.2,0.3,0.4,0.5,0.6,0.7,0.8,0.9,1]  BreakpointsForDimension2=[1:3]  Table=[0.019242,0.038636,0.046717,0.049444,0.048333,0.043384,0.043081,0.045202,0.049242,0.051465,0.05197,0.050556,0.046111,0.040556,0.033081,0.024596,0.015543,0.0059848,-0.0059091,-0.013687,-0.016818]  InternalRulePriority=Speed  RndMeth=Simplest  InputSameDT=on
  n+::Kt-推力系数 : Lookup_n-D  NumberOfTableDimensions=1  BreakpointsForDimension1=[-1,-0.9,-0.8,-0.7,-0.6,-0.5,-0.4,-0.3,-0.2,-0.1,0,0.1,0.2,0.3,0.4,0.5,0.6,0.7,0.8,0.9,1]  BreakpointsForDimension2=[1:3]  Table=[0.082134,0.19766,0.30499,0.32898,0.31256,0.2589,0.25511,0.28226,0.35107,0.3738,0.38,0.36686,0.32645,0.26016,0.18188,0.10423,0.04173,-0.018245,-0.05423,-0.065593,-0.06]  InternalRulePriority=Speed  RndMeth=Simplest  InputSameDT=on
  Kt : Outport
  Kq : Outport  Port=2
  wires:
  J'/1 -> n+::Kt-推力系数/1, n+::Kq-扭矩系数/1
  n+::Kt-推力系数/1 -> Kt/1
  n+::Kq-扭矩系数/1 -> Kq/1

== system propeller/直接转矩控制/船体、水体物理模型/推进器1/螺旋桨模型/螺旋桨工作特性表/If Action Subsystem3 ==
  J' : Inport
  Action Port : ActionPort  ActionPortLabel=else
  n-::Kq-扭矩系数 : Lookup_n-D  NumberOfTableDimensions=1  BreakpointsForDimension1=[-1,-0.9,-0.8,-0.7,-0.6,-0.5,-0.4,-0.3,-0.2,-0.1,0,0.1,0.2,0.3,0.4,0.5,0.6,0.7,0.8,0.9,1]  BreakpointsForDimension2=[1:3]  Table=[0.019242,0.016111,0.010354,-0.00035354,-0.014293,-0.025707,-0.034495,-0.041263,-0.046515,-0.051162,-0.05197,-0.051465,-0.049242,-0.045202,-0.043081,-0.043384,-0.04702,-0.049343,-0.045909,-0.038434,-0.016818]  InternalRulePriority=Speed  RndMeth=Simplest  InputSameDT=on
  n-::Kt-推力系数 : Lookup_n-D  NumberOfTableDimensions=1  BreakpointsForDimension1=[-1,-0.9,-0.8,-0.7,-0.6,-0.5,-0.4,-0.3,-0.2,-0.1,0,0.1,0.2,0.3,0.4,0.5,0.6,0.7,0.8,0.9,1]  BreakpointsForDimension2=[1:3]  Table=[0.082134,0.088952,0.080745,0.052336,-0.020896,-0.090341,-0.16989,-0.25764,-0.32014,-0.34981,-0.35676,-0.35549,-0.33409,-0.29015,-0.25379,-0.24924,-0.30379,-0.32197,-0.2947,-0.21894,-0.06]  InternalRulePriority=Speed  RndMeth=Simplest  InputSameDT=on
  Kt : Outport
  Kq : Outport  Port=2
  wires:
  n-::Kq-扭矩系数/1 -> Kq/1
  n-::Kt-推力系数/1 -> Kt/1
  J'/1 -> n-::Kt-推力系数/1, n-::Kq-扭矩系数/1

== system propeller/直接转矩控制/船体、水体物理模型/推进器1/螺旋桨模型/螺旋桨工作特性表Backup/If Action Subsystem2 ==
  J' : Inport
  Action Port : ActionPort
  n+::Kq-扭矩系数 : Lookup_n-D  NumberOfTableDimensions=1  BreakpointsForDimension1=[-1,-0.9,-0.8,-0.7,-0.6,-0.5,-0.4,-0.3,-0.2,-0.1,0,0.1,0.2,0.3,0.4,0.5,0.6,0.7,0.8,0.9,1]  BreakpointsForDimension2=[1:3]  Table=[0.019242,0.038636,0.046717,0.049444,0.048333,0.043384,0.043081,0.045202,0.049242,0.051465,0.05197,0.050556,0.046111,0.040556,0.033081,0.024596,0.015543,0.0059848,-0.0059091,-0.013687,-0.016818]  InternalRulePriority=Speed  RndMeth=Simplest  InputSameDT=on
  n+::Kt-推力系数 : Lookup_n-D  NumberOfTableDimensions=1  BreakpointsForDimension1=[-1,-0.9,-0.8,-0.7,-0.6,-0.5,-0.4,-0.3,-0.2,-0.1,0,0.1,0.2,0.3,0.4,0.5,0.6,0.7,0.8,0.9,1]  BreakpointsForDimension2=[1:3]  Table=[0.082134,0.19766,0.30499,0.32898,0.31256,0.2589,0.25511,0.28226,0.35107,0.3738,0.38,0.36686,0.32645,0.26016,0.18188,0.10423,0.04173,-0.018245,-0.05423,-0.065593,-0.06]  InternalRulePriority=Speed  RndMeth=Simplest  InputSameDT=on
  Kt : Outport
  Kq : Outport  Port=2
  wires:
  n+::Kq-扭矩系数/1 -> Kq/1
  n+::Kt-推力系数/1 -> Kt/1
  J'/1 -> n+::Kq-扭矩系数/1, n+::Kt-推力系数/1

== system propeller/直接转矩控制/船体、水体物理模型/推进器1/螺旋桨模型/螺旋桨工作特性表Backup/If Action Subsystem3 ==
  J' : Inport
  Action Port : ActionPort
  n-::Kq-扭矩系数 : Lookup_n-D  NumberOfTableDimensions=1  BreakpointsForDimension1=[-1,-0.9,-0.8,-0.7,-0.6,-0.5,-0.4,-0.3,-0.2,-0.1,0,0.1,0.2,0.3,0.4,0.5,0.6,0.7,0.8,0.9,1]  BreakpointsForDimension2=[1:3]  Table=[0.019242,0.016111,0.010354,-0.00035354,-0.014293,-0.025707,-0.034495,-0.041263,-0.046515,-0.051162,-0.05197,-0.051465,-0.049242,-0.045202,-0.043081,-0.043384,-0.04702,-0.049343,-0.045909,-0.038434,-0.016818]  InternalRulePriority=Speed  RndMeth=Simplest  InputSameDT=on
  n-::Kt-推力系数 : Lookup_n-D  NumberOfTableDimensions=1  BreakpointsForDimension1=[-1,-0.9,-0.8,-0.7,-0.6,-0.5,-0.4,-0.3,-0.2,-0.1,0,0.1,0.2,0.3,0.4,0.5,0.6,0.7,0.8,0.9,1]  BreakpointsForDimension2=[1:3]  Table=[0.082134,0.088952,0.080745,0.052336,-0.020896,-0.090341,-0.16989,-0.25764,-0.32014,-0.34981,-0.35676,-0.35549,-0.33409,-0.29015,-0.25379,-0.24924,-0.30379,-0.32197,-0.2947,-0.21894,-0.06]  InternalRulePriority=Speed  RndMeth=Simplest  InputSameDT=on
  Kt : Outport
  Kq : Outport  Port=2
  wires:
  J'/1 -> n-::Kq-扭矩系数/1, n-::Kt-推力系数/1
  n-::Kt-推力系数/1 -> Kt/1
  n-::Kq-扭矩系数/1 -> Kq/1

== system propeller/直接转矩控制/船体、水体物理模型/推进器2/螺旋桨模型/螺旋桨工作特性表/If Action Subsystem2 ==
  J' : Inport
  Action Port : ActionPort  ActionPortLabel=if(u1 > 0)
  n+::Kq-扭矩系数 : Lookup_n-D  NumberOfTableDimensions=1  BreakpointsForDimension1=[-1,-0.9,-0.8,-0.7,-0.6,-0.5,-0.4,-0.3,-0.2,-0.1,0,0.1,0.2,0.3,0.4,0.5,0.6,0.7,0.8,0.9,1]  BreakpointsForDimension2=[1:3]  Table=[0.019242,0.038636,0.046717,0.049444,0.048333,0.043384,0.043081,0.045202,0.049242,0.051465,0.05197,0.050556,0.046111,0.040556,0.033081,0.024596,0.015543,0.0059848,-0.0059091,-0.013687,-0.016818]  InternalRulePriority=Speed  RndMeth=Simplest  InputSameDT=on
  n+::Kt-推力系数 : Lookup_n-D  NumberOfTableDimensions=1  BreakpointsForDimension1=[-1,-0.9,-0.8,-0.7,-0.6,-0.5,-0.4,-0.3,-0.2,-0.1,0,0.1,0.2,0.3,0.4,0.5,0.6,0.7,0.8,0.9,1]  BreakpointsForDimension2=[1:3]  Table=[0.082134,0.19766,0.30499,0.32898,0.31256,0.2589,0.25511,0.28226,0.35107,0.3738,0.38,0.36686,0.32645,0.26016,0.18188,0.10423,0.04173,-0.018245,-0.05423,-0.065593,-0.06]  InternalRulePriority=Speed  RndMeth=Simplest  InputSameDT=on
  Kt : Outport
  Kq : Outport  Port=2
  wires:
  n+::Kq-扭矩系数/1 -> Kq/1
  n+::Kt-推力系数/1 -> Kt/1
  J'/1 -> n+::Kq-扭矩系数/1, n+::Kt-推力系数/1

== system propeller/直接转矩控制/船体、水体物理模型/推进器2/螺旋桨模型/螺旋桨工作特性表/If Action Subsystem3 ==
  J' : Inport
  Action Port : ActionPort  ActionPortLabel=else
  n-::Kq-扭矩系数 : Lookup_n-D  NumberOfTableDimensions=1  BreakpointsForDimension1=[-1,-0.9,-0.8,-0.7,-0.6,-0.5,-0.4,-0.3,-0.2,-0.1,0,0.1,0.2,0.3,0.4,0.5,0.6,0.7,0.8,0.9,1]  BreakpointsForDimension2=[1:3]  Table=[0.019242,0.016111,0.010354,-0.00035354,-0.014293,-0.025707,-0.034495,-0.041263,-0.046515,-0.051162,-0.05197,-0.051465,-0.049242,-0.045202,-0.043081,-0.043384,-0.04702,-0.049343,-0.045909,-0.038434,-0.016818]  InternalRulePriority=Speed  RndMeth=Simplest  InputSameDT=on
  n-::Kt-推力系数 : Lookup_n-D  NumberOfTableDimensions=1  BreakpointsForDimension1=[-1,-0.9,-0.8,-0.7,-0.6,-0.5,-0.4,-0.3,-0.2,-0.1,0,0.1,0.2,0.3,0.4,0.5,0.6,0.7,0.8,0.9,1]  BreakpointsForDimension2=[1:3]  Table=[0.082134,0.088952,0.080745,0.052336,-0.020896,-0.090341,-0.16989,-0.25764,-0.32014,-0.34981,-0.35676,-0.35549,-0.33409,-0.29015,-0.25379,-0.24924,-0.30379,-0.32197,-0.2947,-0.21894,-0.06]  InternalRulePriority=Speed  RndMeth=Simplest  InputSameDT=on
  Kt : Outport
  Kq : Outport  Port=2
  wires:
  J'/1 -> n-::Kq-扭矩系数/1, n-::Kt-推力系数/1
  n-::Kt-推力系数/1 -> Kt/1
  n-::Kq-扭矩系数/1 -> Kq/1

== system propeller/直接转矩控制/船体、水体物理模型/推进器2/螺旋桨模型/螺旋桨工作特性表Backup/If Action Subsystem2 ==
  J' : Inport
  Action Port : ActionPort
  n+::Kq-扭矩系数 : Lookup_n-D  NumberOfTableDimensions=1  BreakpointsForDimension1=[-1,-0.9,-0.8,-0.7,-0.6,-0.5,-0.4,-0.3,-0.2,-0.1,0,0.1,0.2,0.3,0.4,0.5,0.6,0.7,0.8,0.9,1]  BreakpointsForDimension2=[1:3]  Table=[0.019242,0.038636,0.046717,0.049444,0.048333,0.043384,0.043081,0.045202,0.049242,0.051465,0.05197,0.050556,0.046111,0.040556,0.033081,0.024596,0.015543,0.0059848,-0.0059091,-0.013687,-0.016818]  InternalRulePriority=Speed  RndMeth=Simplest  InputSameDT=on
  n+::Kt-推力系数 : Lookup_n-D  NumberOfTableDimensions=1  BreakpointsForDimension1=[-1,-0.9,-0.8,-0.7,-0.6,-0.5,-0.4,-0.3,-0.2,-0.1,0,0.1,0.2,0.3,0.4,0.5,0.6,0.7,0.8,0.9,1]  BreakpointsForDimension2=[1:3]  Table=[0.082134,0.19766,0.30499,0.32898,0.31256,0.2589,0.25511,0.28226,0.35107,0.3738,0.38,0.36686,0.32645,0.26016,0.18188,0.10423,0.04173,-0.018245,-0.05423,-0.065593,-0.06]  InternalRulePriority=Speed  RndMeth=Simplest  InputSameDT=on
  Kt : Outport
  Kq : Outport  Port=2
  wires:
  J'/1 -> n+::Kt-推力系数/1, n+::Kq-扭矩系数/1
  n+::Kt-推力系数/1 -> Kt/1
  n+::Kq-扭矩系数/1 -> Kq/1

== system propeller/直接转矩控制/船体、水体物理模型/推进器2/螺旋桨模型/螺旋桨工作特性表Backup/If Action Subsystem3 ==
  J' : Inport
  Action Port : ActionPort
  n-::Kq-扭矩系数 : Lookup_n-D  NumberOfTableDimensions=1  BreakpointsForDimension1=[-1,-0.9,-0.8,-0.7,-0.6,-0.5,-0.4,-0.3,-0.2,-0.1,0,0.1,0.2,0.3,0.4,0.5,0.6,0.7,0.8,0.9,1]  BreakpointsForDimension2=[1:3]  Table=[0.019242,0.016111,0.010354,-0.00035354,-0.014293,-0.025707,-0.034495,-0.041263,-0.046515,-0.051162,-0.05197,-0.051465,-0.049242,-0.045202,-0.043081,-0.043384,-0.04702,-0.049343,-0.045909,-0.038434,-0.016818]  InternalRulePriority=Speed  RndMeth=Simplest  InputSameDT=on
  n-::Kt-推力系数 : Lookup_n-D  NumberOfTableDimensions=1  BreakpointsForDimension1=[-1,-0.9,-0.8,-0.7,-0.6,-0.5,-0.4,-0.3,-0.2,-0.1,0,0.1,0.2,0.3,0.4,0.5,0.6,0.7,0.8,0.9,1]  BreakpointsForDimension2=[1:3]  Table=[0.082134,0.088952,0.080745,0.052336,-0.020896,-0.090341,-0.16989,-0.25764,-0.32014,-0.34981,-0.35676,-0.35549,-0.33409,-0.29015,-0.25379,-0.24924,-0.30379,-0.32197,-0.2947,-0.21894,-0.06]  InternalRulePriority=Speed  RndMeth=Simplest  InputSameDT=on
  Kt : Outport
  Kq : Outport  Port=2
  wires:
  n-::Kq-扭矩系数/1 -> Kq/1
  n-::Kt-推力系数/1 -> Kt/1
  J'/1 -> n-::Kt-推力系数/1, n-::Kq-扭矩系数/1

== system propeller/直接转矩控制/船速、朝向控制器/推力解算/扭矩有解/If Action Subsystem/无解 ==
  Action Port : ActionPort  ActionPortLabel=if(u1 < 1e-6)
  Constant : Constant  Value=0
  Constant1 : Constant  Value=0
  Mux : Mux  Inputs=2
  Out1 : Outport
  wires:
  Constant/1 -> Mux/1
  Constant1/1 -> Mux/2
  Mux/1 -> Out1/1

== system propeller/直接转矩控制/船速、朝向控制器/推力解算/扭矩有解/If Action Subsystem/有解 ==
  In1 : Inport
  Action Port : ActionPort  ActionPortLabel=else
  F1 : Fcn  Expr=u(1)/cos(u(3)) - u(7)*cos(u(4))/cos(u(3))
  F2 : Fcn  Expr=(u(1)/cos(u(3)) + u(2)/(u(6)*sin(u(5)+u(3))))/(cos(u(4))/cos(u(3)) + sin(u(5)-u(4))/sin(u(5)+u(3)))
  Mux : Mux  Inputs=2
  Mux1 : Mux  Inputs=2
  Out1 : Outport
  wires:
  In1/1 -> Mux1/1, F2/1
  F2/1 -> Mux1/2, Mux/2
  Mux1/1 -> F1/1
  Mux/1 -> Out1/1
  F1/1 -> Mux/1

== system propeller/直接转矩控制/船速、朝向控制器/推力解算/扭矩有解/If Action Subsystem1/无解 ==
  Action Port : ActionPort  ActionPortLabel=if(u1 < 1e-6)
  Constant : Constant  Value=0
  Constant1 : Constant  Value=0
  Mux : Mux  Inputs=2
  Out1 : Outport
  wires:
  Mux/1 -> Out1/1
  Constant1/1 -> Mux/2
  Constant/1 -> Mux/1

== system propeller/直接转矩控制/船速、朝向控制器/推力解算/扭矩有解/If Action Subsystem1/有解 ==
  In1 : Inport
  Action Port : ActionPort  ActionPortLabel=else
  F1 : Fcn  Expr=(u(1)/cos(u(4)) - u(2)/(u(6)*sin(u(5)-u(4))))/(cos(u(3))/cos(u(4)) + sin(u(5)+u(3))/sin(u(5)-u(4)))
  F2 : Fcn  Expr=u(1)/cos(u(4)) - u(7)*cos(u(3))/cos(u(4))
  Mux : Mux  Inputs=2
  Mux1 : Mux  Inputs=2
  Out1 : Outport
  wires:
  F2/1 -> Mux/2
  Mux/1 -> Out1/1
  Mux1/1 -> F2/1
  F1/1 -> Mux/1, Mux1/2
  In1/1 -> F1/1, Mux1/1

== system propeller/直接转矩控制/船速、朝向控制器/舵内缩指令/Subsystem/收敛用推力解算/扭矩无解 ==
  In1 : Inport
  Action Port : ActionPort  ActionPortLabel=if(u1 < 1e-6)
  Mux : Mux  Inputs=2
  只计算前进推力 : Fcn  Expr=u(1)/(cos(u(5)))*0.5
  Out1 : Outport
  wires:
  In1/1 -> 只计算前进推力/1
  只计算前进推力/1 -> Mux/2, Mux/1
  Mux/1 -> Out1/1

== system propeller/直接转矩控制/船速、朝向控制器/舵内缩指令/Subsystem/收敛用推力解算/扭矩有解 ==
  状态输入 : Inport
  Action Port : ActionPort  ActionPortLabel=else
  If : If
  If Action Subsystem : Subsystem  TreatAsAtomicUnit=on
  If Action Subsystem1 : Subsystem  TreatAsAtomicUnit=on
  Merge : Merge
  通解选择 : Fcn  Expr=abs(u(5)+u(3)) - abs(u(5)-u(4))
  推力输出 : Outport
  wires:
  If Action Subsystem/1(推力) -> Merge/1
  If/1 -> If Action Subsystem/Action
  状态输入/1 -> If Action Subsystem1/1(In1), 通解选择/1, If Action Subsystem/1(In1)
  通解选择/1 -> If/1
  If Action Subsystem1/1(推力) -> Merge/2
  If/2 -> If Action Subsystem1/Action
  Merge/1 -> 推力输出/1  "推力输出"

== system propeller/直接转矩控制/船速、朝向控制器/舵朝向指令/Subsystem/收敛用推力解算/扭矩无解 ==
  In1 : Inport
  Action Port : ActionPort  ActionPortLabel=if(u1 < 1e-6)
  Mux : Mux  Inputs=2
  只计算前进推力 : Fcn  Expr=u(1)/(cos(u(5)))*0.5
  Out1 : Outport
  wires:
  Mux/1 -> Out1/1
  只计算前进推力/1 -> Mux/1, Mux/2
  In1/1 -> 只计算前进推力/1

== system propeller/直接转矩控制/船速、朝向控制器/舵朝向指令/Subsystem/收敛用推力解算/扭矩有解 ==
  状态输入 : Inport
  Action Port : ActionPort  ActionPortLabel=else
  If : If
  If Action Subsystem : Subsystem  TreatAsAtomicUnit=on
  If Action Subsystem1 : Subsystem  TreatAsAtomicUnit=on
  Merge : Merge
  通解选择 : Fcn  Expr=abs(u(5)+u(3)) - abs(u(5)-u(4))
  推力输出 : Outport
  wires:
  Merge/1 -> 推力输出/1  "推力输出"
  If/2 -> If Action Subsystem1/Action
  If Action Subsystem1/1(推力) -> Merge/2
  通解选择/1 -> If/1
  状态输入/1 -> If Action Subsystem/1(In1), 通解选择/1, If Action Subsystem1/1(In1)
  If/1 -> If Action Subsystem/Action
  If Action Subsystem/1(推力) -> Merge/1

== system propeller/直接转矩控制/船速、朝向控制器/舵内缩指令/Subsystem/收敛用推力解算/扭矩有解/If Action Subsystem ==
  In1 : Inport
  Action Port : ActionPort  ActionPortLabel=if(u1 > 0)
  Abs : Abs
  If : If  IfExpression=u1 < 1e-6
  Merge : Merge
  无解 : Subsystem  TreatAsAtomicUnit=on
  有解 : Subsystem  TreatAsAtomicUnit=on
  通解分母 : Fcn  Expr=(cos(u(4))/cos(u(3)) + sin(u(5)-u(4))/sin(u(5)+u(3)))
  推力 : Outport
  wires:
  通解分母/1 -> Abs/1
  In1/1 -> 有解/1(In1), 通解分母/1
  Abs/1 -> If/1
  If/1 -> 无解/Action
  If/2 -> 有解/Action
  Merge/1 -> 推力/1
  无解/1(Out1) -> Merge/1
  有解/1(Out1) -> Merge/2

== system propeller/直接转矩控制/船速、朝向控制器/舵内缩指令/Subsystem/收敛用推力解算/扭矩有解/If Action Subsystem1 ==
  In1 : Inport
  Action Port : ActionPort  ActionPortLabel=else
  Abs : Abs
  If : If  IfExpression=u1 < 1e-6
  Merge : Merge
  无解 : Subsystem  TreatAsAtomicUnit=on
  有解 : Subsystem  TreatAsAtomicUnit=on
  通解分母 : Fcn  Expr=(cos(u(3))/cos(u(4)) + sin(u(5)+u(3))/sin(u(5)-u(4)))
  推力 : Outport
  wires:
  有解/1(Out1) -> Merge/2
  无解/1(Out1) -> Merge/1
  Merge/1 -> 推力/1
  If/2 -> 有解/Action
  If/1 -> 无解/Action
  Abs/1 -> If/1
  In1/1 -> 通解分母/1, 有解/1(In1)
  通解分母/1 -> Abs/1

== system propeller/直接转矩控制/船速、朝向控制器/舵朝向指令/Subsystem/收敛用推力解算/扭矩有解/If Action Subsystem ==
  In1 : Inport
  Action Port : ActionPort  ActionPortLabel=if(u1 > 0)
  Abs : Abs
  If : If  IfExpression=u1 < 1e-6
  Merge : Merge
  无解 : Subsystem  TreatAsAtomicUnit=on
  有解 : Subsystem  TreatAsAtomicUnit=on
  通解分母 : Fcn  Expr=(cos(u(4))/cos(u(3)) + sin(u(5)-u(4))/sin(u(5)+u(3)))
  推力 : Outport
  wires:
  有解/1(Out1) -> Merge/2
  无解/1(Out1) -> Merge/1
  Merge/1 -> 推力/1
  If/2 -> 有解/Action
  If/1 -> 无解/Action
  Abs/1 -> If/1
  In1/1 -> 通解分母/1, 有解/1(In1)
  通解分母/1 -> Abs/1

== system propeller/直接转矩控制/船速、朝向控制器/舵朝向指令/Subsystem/收敛用推力解算/扭矩有解/If Action Subsystem1 ==
  In1 : Inport
  Action Port : ActionPort  ActionPortLabel=else
  Abs : Abs
  If : If  IfExpression=u1 < 1e-6
  Merge : Merge
  无解 : Subsystem  TreatAsAtomicUnit=on
  有解 : Subsystem  TreatAsAtomicUnit=on
  通解分母 : Fcn  Expr=(cos(u(3))/cos(u(4)) + sin(u(5)+u(3))/sin(u(5)-u(4)))
  推力 : Outport
  wires:
  通解分母/1 -> Abs/1
  In1/1 -> 有解/1(In1), 通解分母/1
  Abs/1 -> If/1
  If/1 -> 无解/Action
  If/2 -> 有解/Action
  Merge/1 -> 推力/1
  无解/1(Out1) -> Merge/1
  有解/1(Out1) -> Merge/2

== system propeller/直接转矩控制/船速、朝向控制器/舵内缩指令/Subsystem/收敛用推力解算/扭矩有解/If Action Subsystem/无解 ==
  Action Port : ActionPort  ActionPortLabel=if(u1 < 1e-6)
  Constant : Constant  Value=0
  Constant1 : Constant  Value=0
  Mux : Mux  Inputs=2
  Out1 : Outport
  wires:
  Constant/1 -> Mux/1
  Constant1/1 -> Mux/2
  Mux/1 -> Out1/1

== system propeller/直接转矩控制/船速、朝向控制器/舵内缩指令/Subsystem/收敛用推力解算/扭矩有解/If Action Subsystem/有解 ==
  In1 : Inport
  Action Port : ActionPort  ActionPortLabel=else
  F1 : Fcn  Expr=u(1)/cos(u(3)) - u(7)*cos(u(4))/cos(u(3))
  F2 : Fcn  Expr=(u(1)/cos(u(3)) + u(2)/(u(6)*sin(u(5)+u(3))))/(cos(u(4))/cos(u(3)) + sin(u(5)-u(4))/sin(u(5)+u(3)))
  Mux : Mux  Inputs=2
  Mux1 : Mux  Inputs=2
  Out1 : Outport
  wires:
  In1/1 -> Mux1/1, F2/1
  F2/1 -> Mux1/2, Mux/2
  Mux1/1 -> F1/1
  Mux/1 -> Out1/1
  F1/1 -> Mux/1

== system propeller/直接转矩控制/船速、朝向控制器/舵内缩指令/Subsystem/收敛用推力解算/扭矩有解/If Action Subsystem1/无解 ==
  Action Port : ActionPort  ActionPortLabel=if(u1 < 1e-6)
  Constant : Constant  Value=0
  Constant1 : Constant  Value=0
  Mux : Mux  Inputs=2
  Out1 : Outport
  wires:
  Mux/1 -> Out1/1
  Constant1/1 -> Mux/2
  Constant/1 -> Mux/1

== system propeller/直接转矩控制/船速、朝向控制器/舵内缩指令/Subsystem/收敛用推力解算/扭矩有解/If Action Subsystem1/有解 ==
  In1 : Inport
  Action Port : ActionPort  ActionPortLabel=else
  F1 : Fcn  Expr=(u(1)/cos(u(4)) - u(2)/(u(6)*sin(u(5)-u(4))))/(cos(u(3))/cos(u(4)) + sin(u(5)+u(3))/sin(u(5)-u(4)))
  F2 : Fcn  Expr=u(1)/cos(u(4)) - u(7)*cos(u(3))/cos(u(4))
  Mux : Mux  Inputs=2
  Mux1 : Mux  Inputs=2
  Out1 : Outport
  wires:
  F2/1 -> Mux/2
  Mux/1 -> Out1/1
  Mux1/1 -> F2/1
  F1/1 -> Mux/1, Mux1/2
  In1/1 -> F1/1, Mux1/1

== system propeller/直接转矩控制/船速、朝向控制器/舵朝向指令/Subsystem/收敛用推力解算/扭矩有解/If Action Subsystem/无解 ==
  Action Port : ActionPort  ActionPortLabel=if(u1 < 1e-6)
  Constant : Constant  Value=0
  Constant1 : Constant  Value=0
  Mux : Mux  Inputs=2
  Out1 : Outport
  wires:
  Mux/1 -> Out1/1
  Constant1/1 -> Mux/2
  Constant/1 -> Mux/1

== system propeller/直接转矩控制/船速、朝向控制器/舵朝向指令/Subsystem/收敛用推力解算/扭矩有解/If Action Subsystem/有解 ==
  In1 : Inport
  Action Port : ActionPort  ActionPortLabel=else
  F1 : Fcn  Expr=u(1)/cos(u(3)) - u(7)*cos(u(4))/cos(u(3))
  F2 : Fcn  Expr=(u(1)/cos(u(3)) + u(2)/(u(6)*sin(u(5)+u(3))))/(cos(u(4))/cos(u(3)) + sin(u(5)-u(4))/sin(u(5)+u(3)))
  Mux : Mux  Inputs=2
  Mux1 : Mux  Inputs=2
  Out1 : Outport
  wires:
  F1/1 -> Mux/1
  Mux/1 -> Out1/1
  Mux1/1 -> F1/1
  F2/1 -> Mux/2, Mux1/2
  In1/1 -> F2/1, Mux1/1

== system propeller/直接转矩控制/船速、朝向控制器/舵朝向指令/Subsystem/收敛用推力解算/扭矩有解/If Action Subsystem1/无解 ==
  Action Port : ActionPort  ActionPortLabel=if(u1 < 1e-6)
  Constant : Constant  Value=0
  Constant1 : Constant  Value=0
  Mux : Mux  Inputs=2
  Out1 : Outport
  wires:
  Constant/1 -> Mux/1
  Constant1/1 -> Mux/2
  Mux/1 -> Out1/1

== system propeller/直接转矩控制/船速、朝向控制器/舵朝向指令/Subsystem/收敛用推力解算/扭矩有解/If Action Subsystem1/有解 ==
  In1 : Inport
  Action Port : ActionPort  ActionPortLabel=else
  F1 : Fcn  Expr=(u(1)/cos(u(4)) - u(2)/(u(6)*sin(u(5)-u(4))))/(cos(u(3))/cos(u(4)) + sin(u(5)+u(3))/sin(u(5)-u(4)))
  F2 : Fcn  Expr=u(1)/cos(u(4)) - u(7)*cos(u(3))/cos(u(4))
  Mux : Mux  Inputs=2
  Mux1 : Mux  Inputs=2
  Out1 : Outport
  wires:
  In1/1 -> Mux1/1, F1/1
  F1/1 -> Mux1/2, Mux/1
  Mux1/1 -> F2/1
  Mux/1 -> Out1/1
  F2/1 -> Mux/2
